simulink model "main"  (Simulink 3.00)
libraries: mathlib x4, genlib x3, speclib x1, matrixlib x1, arclib x1

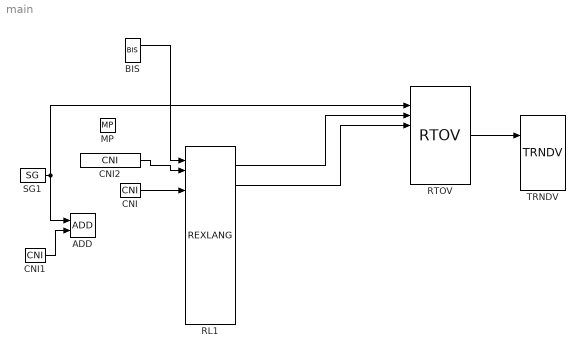
== system main ==
  ADD : mathlib/ADD
  BIS : genlib/BIS  Y0=off  t1=1  t2=2  t3=0  t4=4  t5=5  t6=6  t7=7  t8=8  RPT=on
  CNI : mathlib/CNI  icn=1
  CNI1 : mathlib/CNI  icn=32767
  CNI2 : mathlib/CNI  icn=0xABCD
  MP : genlib/MP  pwidth=1  BSTATE=off  RPTF=off
  RL1 : speclib/REXLANG  srcname=rl1.stl  srctype=1: STL  debug=1: No check  fname=/dev/spidev0.0  stack=0  strs=0  p0=0x638
  RTOV : matrixlib/RTOV  capacity=8  offset=0  n=8  Type=8: Double
  SG1 : genlib/SG  isig=1: SINE  amp=32767  freq=0.1  phase=0.0000000E+000  ifrunit=1: Hz  iphunit=1: degrees
  TRNDV : arclib/TRNDV  n=8  l=10000  btype=8: Double  pfac=1  afac=0  arc=0  id=1  Title=Trend Title
  wires:
  BIS/1 -> RL1/2
  CNI/1 -> RL1/5
  CNI1/1 -> ADD/2
  CNI2/1 -> RL1/3
  RL1/2 -> RTOV/3
  RL1/4 -> RTOV/4
  RTOV/1 -> TRNDV/1
  SG1/1 -> ADD/1, RTOV/2
